simulink model "hdlcoder_sobel_video_stream"  (R2017b)
settings: Solver=FixedStepDiscrete  StartTime=0.0  StopTime=Ts_240p*5  RelTol=1e-3
InitFcn:
  | Ts = 1e-3;
  | Ts_240p = 402*324*Ts;
undefined symbols (not defined in the file): Rec, SDTV
libraries: hdlsllib x8, visionhdlio x2, simulink x2, visionhdlconversions x1, visionhdlanalysis x1, dspvision x1
settings Model: DataTypeOverride=Off  ModifiedByFormat=The MathWorks Inc.  Creator=The MathWorks, Inc.  LastModifiedBy=The MathWorks Inc.
settings DataIOCC: LimitDataPoints=on  SaveFormat=Array  SaveOutput=off  SaveTime=off
settings OptimizationCC: BlockReduction=off  ConditionallyExecuteInputs=off  DefaultParameterBehavior=Inlined  LifeSpan=inf
settings DebuggingCC: AlgebraicLoopMsg=error  SolverPrmCheckMsg=warning  SingleTaskRateTransMsg=error  ParameterPrecisionLossMsg=none  AllowSymbolicDim=off  SFUnexpectedBacktrackingDiag=warning  SFNoUnconditionalDefaultTransitionDiag=warning  SFExecutionAtInitializationDiag=none  IntegerSaturationMsg=none
settings HardwareCC: ProdBitPerPointer=32  ProdBitPerSizeT=32  ProdBitPerPtrDiffT=32  ProdLargestAtomicFloat=None  ProdIntDivRoundTo=Undefined  ProdEndianess=Unspecified  ProdWordSize=32  ProdHWDeviceType=ASIC/FPGA->ASIC/FPGA  ProdEqTarget=off
settings ModelReferenceCC: PropagateSignalLabelsOutOfModel=off
settings CodeAppCC: StateflowObjectComments=on
settings GRTTargetCC: TargetLangStandard=C89/C90 (ANSI)  GeneratePreprocessorConditionals=Disable all
settings ConfigComp: CovMetricSettings=dw  CovHtmlReporting=on  CovSaveCumulativeToWorkspaceVar=on  CovSaveSingleToWorkspaceVar=on  CovShowResultsExplorer=off  CovExternalEMLEnable=off  CovSFcnEnable=off

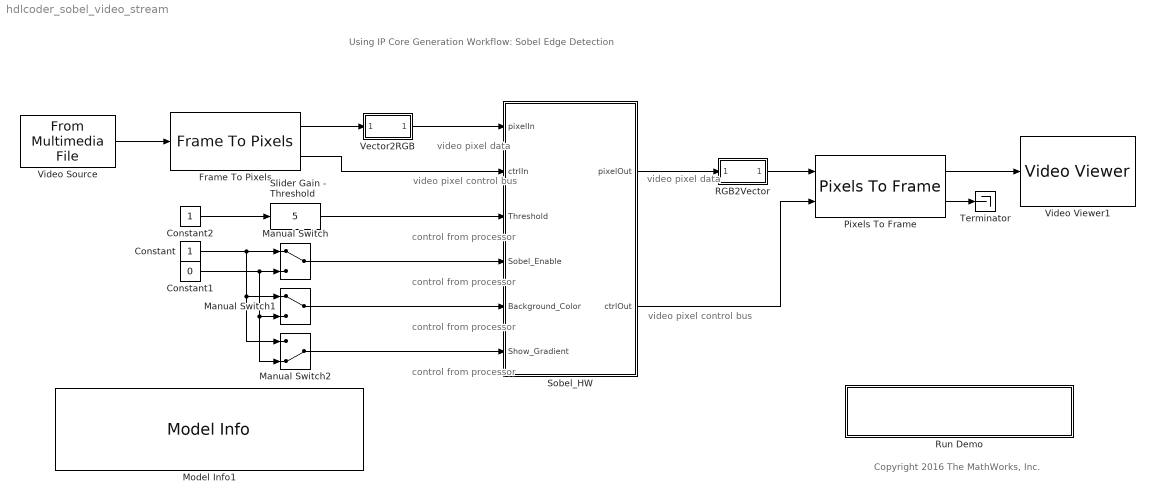
== system hdlcoder_sobel_video_stream ==
  note: control from processor
  note: video pixel data
  note: Copyright 2016 The MathWorks, Inc.
  note: Using IP Core Generation Workflow: Sobel Edge Detection
  note: video pixel control bus
  note: control from processor
  note: control from processor
  note: control from processor
  note: video pixel data
  note: video pixel control bus
  Constant : Constant  OutDataTypeStr=boolean  SampleTime=Ts
  Constant1 : Constant  Value=0  OutDataTypeStr=boolean  SampleTime=Ts
  Constant2 : Constant  OutDataTypeStr=uint8  SampleTime=Ts
  Frame To Pixels : visionhdlio/Frame To Pixels  NumComponents=3  VideoFormat=240p  ActivePixelsPerLine=32  ActiveVideoLines=18  TotalPixelsPerLine=42  TotalVideoLines=28  StartingActiveLine=6  FrontPorch=5  SampleTime=0
      settings: SourceProductName=Vision HDL Toolbox  SourceProductBaseCode=VT
  Manual Switch : ManualSwitch
  Manual Switch1 : ManualSwitch
  Manual Switch2 : ManualSwitch  CurrentSetting=0
  Model Info1 : simulink/Model-Wide Utilities/Model Info  Frame=on  DisplayStringWithTags=|  HorizontalTextAlignment=Left  LeftAlignmentValue=0.02
      | This example shows how to use HDL Coder to
      | generate a custom IP core which perform Sobel
      | edge detection processing on streaming video.
      | 
      | In MATLAB, type the following:
      |   hdladvisor('hdlcoder_sobel_video_stream/Sobel_HW')
  Pixels To Frame : visionhdlio/Pixels To Frame  NumComponents=3  VideoFormat=240p  ActivePixelsPerLine=32  ActiveVideoLines=18  TotalPixelsPerLine=42  TotalVideoLines=28
      settings: SourceProductName=Vision HDL Toolbox  SourceProductBaseCode=VT
  RGB2Vector : Subsystem
  Run Demo : Subsystem
      settings: OpenFcn=hdladvisor([bdroot, '/Sobel_HW'])
      mask Display: disp('Launch HDL Workflow Advisor')
  Slider Gain - Threshold : simulink/Math Operations/Slider Gain  gain=5  low=0  high=100
  Sobel_HW : Subsystem  TreatAsAtomicUnit=on
  Terminator : Terminator
  Vector2RGB : Subsystem
  Video Source : dspvision/From Multimedia File  inputFilename=rhinos.avi  loop=on  numPlays=inf  outputStreams=Video only  videoDataType=uint8  audioDataType=int16  inheritSampleTime=off  userDefinedSampleTime=Ts_240p  noAudioOutput=off  isIntensityVideo=off  fourcc=RGB  colorVideoFormat=One multidimensional signal  outputEOF=off  dataOrg=Column-major  audioFrameSize=1024  computeAudioFrameSize=off  outSamplingMode=Sample based
      settings: SourceProductBaseCode=VP
  Video Viewer1 : VideoViewer  FigPos=[1477 563 410 300]
  wires:
  Pixels To Frame/2 -> Terminator/1
  Pixels To Frame/1 -> Video Viewer1/1
  Manual Switch/1 -> Sobel_HW/4(Sobel_Enable)
  Constant/1 -> Manual Switch2/1, Manual Switch1/1, Manual Switch/1
  Constant1/1 -> Manual Switch2/2, Manual Switch1/2, Manual Switch/2
  Vector2RGB/1(RGB) -> Sobel_HW/1(pixelIn)
  Sobel_HW/1(pixelOut) -> RGB2Vector/1(RGB)
  Video Source/1 -> Frame To Pixels/1
  Frame To Pixels/1 -> Vector2RGB/1(RGBVector)
  Sobel_HW/2(ctrlOut) -> Pixels To Frame/2
  Manual Switch1/1 -> Sobel_HW/5(Background_Color)
  Manual Switch2/1 -> Sobel_HW/6(Show_Gradient)
  Constant2/1 -> Slider Gain - Threshold/1
  Slider Gain - Threshold/1 -> Sobel_HW/3(Threshold)
  Frame To Pixels/2 -> Sobel_HW/2(ctrlIn)
  RGB2Vector/1(RGBVector) -> Pixels To Frame/1

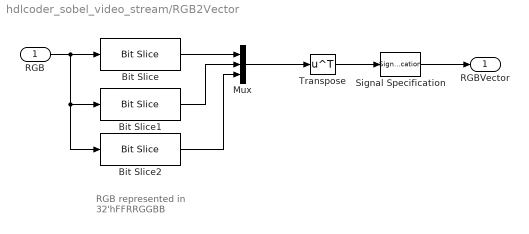
== system hdlcoder_sobel_video_stream/RGB2Vector ==
  note: RGB represented in
      | 32'hFFRRGGBB
  RGB : Inport
  Bit Slice : hdlsllib/HDL Operations/Bit Slice  lidx=23  ridx=16
      settings: SourceProductName=HDL Coder  SourceProductBaseCode=HD
  Bit Slice1 : hdlsllib/HDL Operations/Bit Slice  lidx=15  ridx=8
      settings: SourceProductName=HDL Coder  SourceProductBaseCode=HD
  Bit Slice2 : hdlsllib/HDL Operations/Bit Slice  lidx=7  ridx=0
      settings: SourceProductName=HDL Coder  SourceProductBaseCode=HD
  Mux : Mux  Inputs=3
  Signal Specification : SignalSpecification
  Transpose : Math  Operator=transpose  SaturateOnIntegerOverflow=on
  RGBVector : Outport
  wires:
  Mux/1 -> Transpose/1
  Bit Slice/1 -> Mux/1
  Bit Slice2/1 -> Mux/3
  Bit Slice1/1 -> Mux/2
  RGB/1 -> Bit Slice2/1, Bit Slice1/1, Bit Slice/1
  Transpose/1 -> Signal Specification/1
  Signal Specification/1 -> RGBVector/1

== system hdlcoder_sobel_video_stream/Run Demo ==

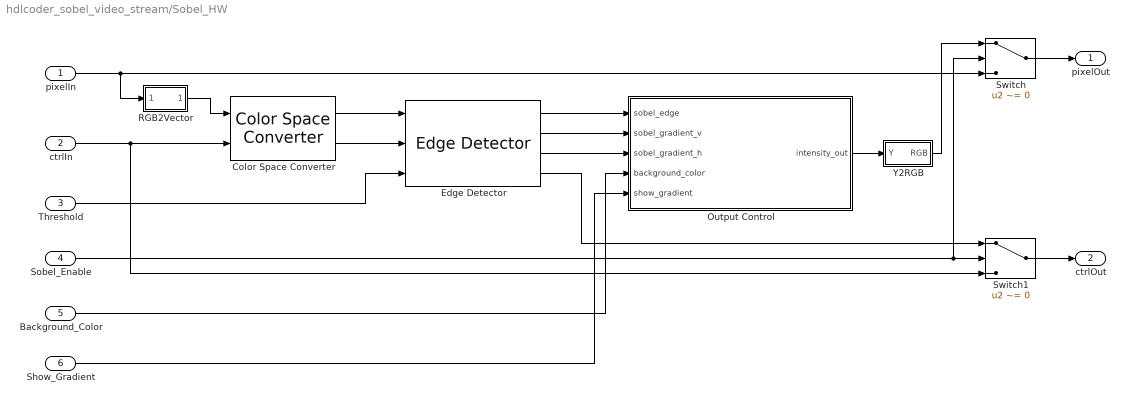
== system hdlcoder_sobel_video_stream/Sobel_HW ==
  pixelIn : Inport
  ctrlIn : Inport  Port=2
  Threshold : Inport  Port=3
  Sobel_Enable : Inport  Port=4
  Background_Color : Inport  Port=5
  Show_Gradient : Inport  Port=6
  Color Space Converter : visionhdlconversions/Color Space Converter  Conversion=RGB to intensity  ConversionStandard=Rec. 601 (SDTV)  ScanningStandard=1250/50/2:1  SimulateUsing=Code generation
      settings: SourceProductName=Vision HDL Toolbox  SourceProductBaseCode=VT
  Edge Detector : visionhdlanalysis/Edge Detector  Method=Sobel  BinaryImageOutputPort=on  GradientComponentOutputPorts=on  ThresholdSource=Input port  Threshold=20  LineBufferSize=2048  SimulateUsing=Code generation  roundingMode=Floor  overflowMode=off  GradientMin=[]  GradientMax=[]
      settings: SourceProductName=Vision HDL Toolbox  SourceProductBaseCode=VT
  Output Control : MATLAB Function  TreatAsAtomicUnit=on
  RGB2Vector : Subsystem
  Switch : Switch  Criteria=u2 ~= 0
  Switch1 : Switch  Criteria=u2 ~= 0
  Y2RGB : Subsystem
  pixelOut : Outport
  ctrlOut : Outport  Port=2
  wires:
  ctrlIn/1 -> Color Space Converter/2, Switch1/3
  Edge Detector/4 -> Switch1/1
  Switch1/1 -> ctrlOut/1
  pixelIn/1 -> Switch/3, RGB2Vector/1(RGB)
  Color Space Converter/1 -> Edge Detector/1
  Color Space Converter/2 -> Edge Detector/2
  Y2RGB/1(RGB) -> Switch/1
  Switch/1 -> pixelOut/1
  RGB2Vector/1(RGBVector) -> Color Space Converter/1
  Sobel_Enable/1 -> Switch/2, Switch1/2
  Threshold/1 -> Edge Detector/3
  Output Control/1(intensity_out) -> Y2RGB/1(Y)
  Edge Detector/1 -> Output Control/1(sobel_edge)
  Edge Detector/2 -> Output Control/2(sobel_gradient_v)
  Edge Detector/3 -> Output Control/3(sobel_gradient_h)
  Background_Color/1 -> Output Control/4(background_color)
  Show_Gradient/1 -> Output Control/5(show_gradient)

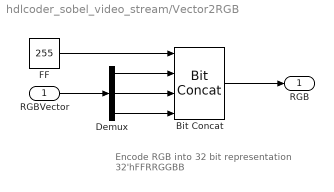
== system hdlcoder_sobel_video_stream/Vector2RGB ==
  note: Encode RGB into 32 bit representation
      | 32'hFFRRGGBB
  RGBVector : Inport
  Bit Concat : hdlsllib/HDL Operations/Bit Concat  numInputs=4
      settings: SourceProductName=HDL Coder  SourceProductBaseCode=HD
  Demux : Demux  Outputs=3
  FF : Constant  Value=255  OutDataTypeStr=uint8  SampleTime=Ts
  RGB : Outport
  wires:
  Bit Concat/1 -> RGB/1
  RGBVector/1 -> Demux/1
  FF/1 -> Bit Concat/1
  Demux/1 -> Bit Concat/2
  Demux/2 -> Bit Concat/3
  Demux/3 -> Bit Concat/4

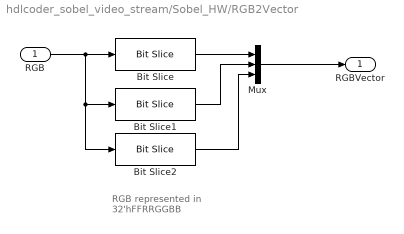
== system hdlcoder_sobel_video_stream/Sobel_HW/RGB2Vector ==
  note: RGB represented in
      | 32'hFFRRGGBB
  RGB : Inport
  Bit Slice : hdlsllib/HDL Operations/Bit Slice  lidx=23  ridx=16
      settings: SourceProductName=HDL Coder  SourceProductBaseCode=HD
  Bit Slice1 : hdlsllib/HDL Operations/Bit Slice  lidx=15  ridx=8
      settings: SourceProductName=HDL Coder  SourceProductBaseCode=HD
  Bit Slice2 : hdlsllib/HDL Operations/Bit Slice  lidx=7  ridx=0
      settings: SourceProductName=HDL Coder  SourceProductBaseCode=HD
  Mux : Mux  Inputs=3
  RGBVector : Outport
  wires:
  Bit Slice/1 -> Mux/1
  Bit Slice2/1 -> Mux/3
  Bit Slice1/1 -> Mux/2
  RGB/1 -> Bit Slice2/1, Bit Slice1/1, Bit Slice/1
  Mux/1 -> RGBVector/1

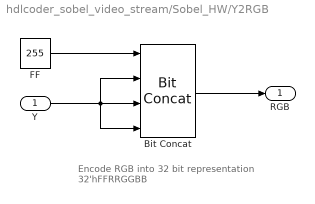
== system hdlcoder_sobel_video_stream/Sobel_HW/Y2RGB ==
  note: Encode RGB into 32 bit representation
      | 32'hFFRRGGBB
  Y : Inport
  Bit Concat : hdlsllib/HDL Operations/Bit Concat  numInputs=4
      settings: SourceProductName=HDL Coder  SourceProductBaseCode=HD
  FF : Constant  Value=255  OutDataTypeStr=uint8  SampleTime=Ts
  RGB : Outport
  wires:
  Bit Concat/1 -> RGB/1
  FF/1 -> Bit Concat/1
  Y/1 -> Bit Concat/4, Bit Concat/2, Bit Concat/3

== matlab function hdlcoder_sobel_video_stream/Sobel_HW/Output Control ==
  data: sobel_edge input boolean; sobel_gradient_v input; sobel_gradient_h input; intensity_out output; background_color input boolean; show_gradient input boolean
function intensity_out = OutputControl(sobel_edge, sobel_gradient_v, sobel_gradient_h, background_color, show_gradient)
% display image based on the control ports

black = fi(0, 0, 8, 0);
white = fi(255, 0, 8, 0);

if show_gradient
    intensity_out = fi(sobel_gradient_v*sobel_gradient_v + sobel_gradient_h*sobel_gradient_h, 0, 8, 0);
else
    if background_color
        % background_color = 1, background is black
        if sobel_edge
            intensity_out = white;
        else
            intensity_out = black;
        end
    else
        % background_color = 0, background is white
        if sobel_edge
            intensity_out = black;
        else
            intensity_out = white;
        end
    end
end
